simulink model "simulink7"  (R2017a)
settings: Solver=ode45  StartTime=0.0  StopTime=5.0  RelTol=1e-3  EnableMultiTasking=on
libraries: cstblocks x3
settings Model: Creator=NAFIZ  LastModifiedBy=ziaba
settings DataIOCC: LimitDataPoints=on  SaveFormat=Array
settings OptimizationCC: LifeSpan=inf
settings DebuggingCC: UnderspecifiedInitializationDetection=Classic  MergeDetectMultiDrivingBlocksExec=none  SolverPrmCheckMsg=warning  StateNameClashWarn=warning  SFUnexpectedBacktrackingDiag=warning  SFNoUnconditionalDefaultTransitionDiag=warning  SFExecutionAtInitializationDiag=none
settings HardwareCC: ProdBitPerPointer=32  ProdBitPerSizeT=32  ProdBitPerPtrDiffT=32  ProdLargestAtomicFloat=None  ProdIntDivRoundTo=Undefined  ProdEndianess=Unspecified  ProdWordSize=32  ProdHWDeviceType=32-bit Generic
settings ModelReferenceCC: PropagateSignalLabelsOutOfModel=off
settings GRTTargetCC: TargetLangStandard=C89/C90 (ANSI)  GeneratePreprocessorConditionals=Disable all
settings ConfigComp: CovMetricSettings=dw  CovHtmlReporting=on  CovSaveCumulativeToWorkspaceVar=on  CovSaveSingleToWorkspaceVar=on  CovExternalEMLEnable=off

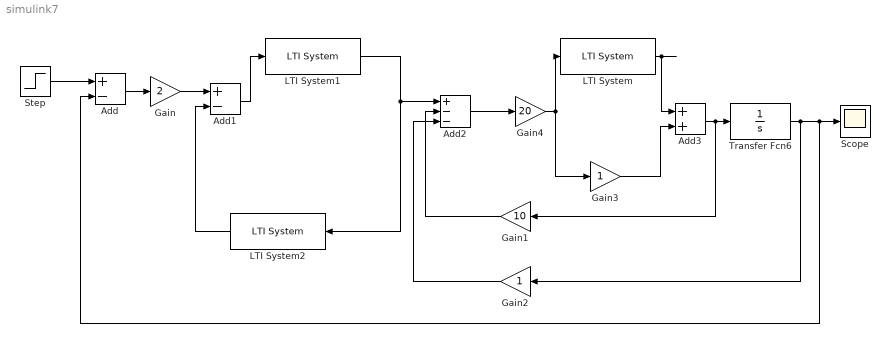
== system simulink7 ==
  Add : Sum  Inputs=+-
  Add1 : Sum  Inputs=+-
  Add2 : Sum  Inputs=+--
  Add3 : Sum
  Gain : Gain  Gain=2
  Gain1 : Gain  Gain=10
  Gain2 : Gain
  Gain3 : Gain
  Gain4 : Gain  Gain=20
  LTI System : cstblocks/LTI System  sys=tf([20 20 1],[1 1 0])  IC=[]
  LTI System1 : cstblocks/LTI System  sys=tf([20 400],[1 0 5])  IC=[]
  LTI System2 : cstblocks/LTI System  sys=tf(3,[1 2 5])  IC=[]
  Scope : Scope
  Step : Step  SampleTime=0
  Transfer Fcn6 : TransferFcn  Denominator=[1 0]
  wires:
  Step/1 -> Add/1
  Add/1 -> Gain/1
  Gain/1 -> Add1/1
  Gain1/1 -> Add2/2
  Gain2/1 -> Add2/3
  Gain3/1 -> Add3/2
  Add3/1 -> Gain1/1, Transfer Fcn6/1
  Transfer Fcn6/1 -> Gain2/1, Add/2, Scope/1
  Add2/1 -> Gain4/1
  Gain4/1 -> Gain3/1, LTI System/1
  Add1/1 -> LTI System1/1
  LTI System2/1 -> Add1/2
  LTI System1/1 -> LTI System2/1, Add2/1
  LTI System/1 -> Add3/1
